simulink model "EDS"  (R2020a)
settings: Solver=VariableStepAuto  StartTime=0.0  StopTime=10.0  RelTol=1e-3
undefined symbols (not defined in the file): magnitude
libraries: simulink x2
settings Model: Creator=Administrator  LastModifiedBy=Administrator

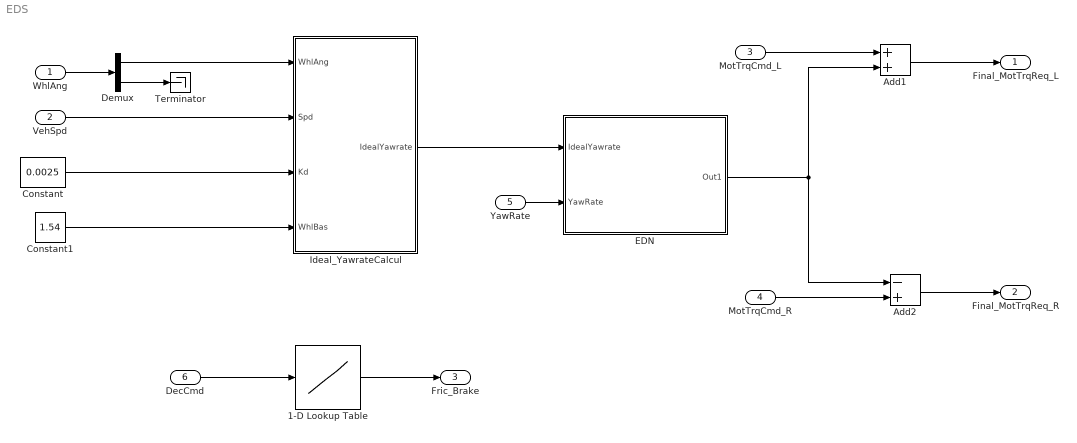
== system EDS ==
  WhlAng : Inport
  VehSpd : Inport  Port=2
  MotTrqCmd_L : Inport  Port=3
  MotTrqCmd_R : Inport  Port=4
  YawRate : Inport  Port=5
  DecCmd : Inport  Port=6
  1-D Lookup Table : Lookup_n-D  NumberOfTableDimensions=1  BreakpointsForDimension1=[0 , 0.2,0.4,0.6,0.8,1.0]  Table=[0 , 0.2,0.4,0.6,0.8,1.0]*60  InternalRulePriority=Speed  RndMeth=Simplest  InputSameDT=on
  Add1 : Sum
  Add2 : Sum  Inputs=-+
  Constant : Constant  Value=0.0025
  Constant1 : Constant  Value=1.54
  Demux : Demux  Outputs=2
  EDN : Subsystem
  Ideal_YawrateCalcul : Subsystem
  Terminator : Terminator
  Final_MotTrqReq_L : Outport
  Final_MotTrqReq_R : Outport  Port=2
  Fric_Brake : Outport  Port=3
  wires:
  WhlAng/1 -> Demux/1
  Demux/2 -> Terminator/1
  VehSpd/1 -> Ideal_YawrateCalcul/2(Spd)
  YawRate/1 -> EDN/2(YawRate)
  Add2/1 -> Final_MotTrqReq_R/1
  EDN/1(Out1) -> Add1/2, Add2/1
  MotTrqCmd_R/1 -> Add2/2
  Add1/1 -> Final_MotTrqReq_L/1
  MotTrqCmd_L/1 -> Add1/1
  Demux/1 -> Ideal_YawrateCalcul/1(WhlAng)
  Constant/1 -> Ideal_YawrateCalcul/3(Kd)
  Constant1/1 -> Ideal_YawrateCalcul/4(WhlBas)
  Ideal_YawrateCalcul/1(IdealYawrate) -> EDN/1(IdealYawrate)
  DecCmd/1 -> 1-D Lookup Table/1
  1-D Lookup Table/1 -> Fric_Brake/1

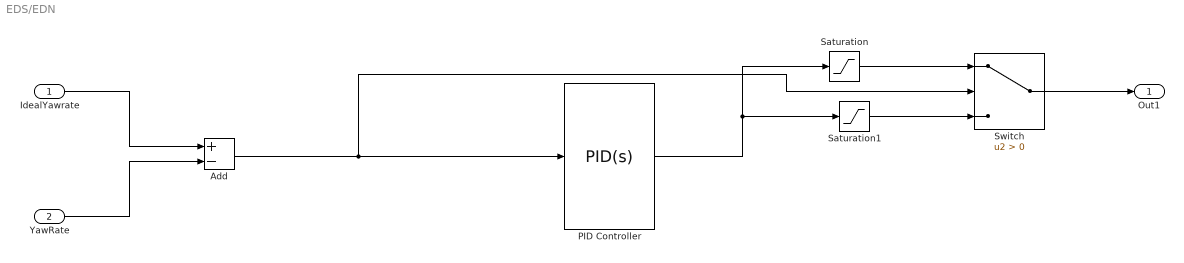
== system EDS/EDN ==
  IdealYawrate : Inport
  YawRate : Inport  Port=2
  Add : Sum  Inputs=+-
  PID Controller : simulink/Continuous/PID Controller  Controller=PID  Form=Parallel  TimeDomain=Continuous-time  UseExternalTs=off  SampleTime=-1  IntegratorMethod=Forward Euler  FilterMethod=Forward Euler  ControllerParametersSource=internal  P=2  I=1  D=0  UseFilter=on  N=100  TunerSelectOption=Transfer Function Based (PID Tuner App)  InitialConditionSource=internal  InitialConditionForIntegrator=0  InitialConditionForFilter=0  DifferentiatorICPrevScaledInput=0  ExternalReset=none  TrackingMode=off  Kt=1  LimitOutput=on  UpperSaturationLimit=30  LowerSaturationLimit=-30  LinearizeAsGain=on  AntiWindupMode=none  Kb=1  SaturateOnIntegerOverflow=on  POutMin=[]  POutMax=[]  IOutMin=[]  IOutMax=[]  DOutMin=[]  DOutMax=[]  NOutMin=[]  NOutMax=[]  SumOutMin=[]  SumOutMax=[]  SaturationOutMin=[]  SaturationOutMax=[]  PParamMin=[]  PParamMax=[]  IParamMin=[]  IParamMax=[]  DParamMin=[]  DParamMax=[]  NParamMin=[]  NParamMax=[]  KbParamMin=[]  KbParamMax=[]  KtParamMin=[]  KtParamMax=[]  KbOutMin=[]  KbOutMax=[]  KtOutMin=[]  KtOutMax=[]  IntegratorOutMin=[]  IntegratorOutMax=[]  FilterOutMin=[]  FilterOutMax=[]  SumI1OutMin=[]  SumI1OutMax=[]  SumI2OutMin=[]  SumI2OutMax=[]  SumI3OutMin=[]  SumI3OutMax=[]  SumI4OutMin=[]  SumI4OutMax=[]  SumDOutMin=[]  SumDOutMax=[]  DifferentiatorOutMin=[]  DifferentiatorOutMax=[]  FilterDiffOutCoefMin=[]  FilterDiffOutCoefMax=[]  ReciprocalOutMin=[]  ReciprocalOutMax=[]  SumDenOutMin=[]  SumDenOutMax=[]  SumNumOutMin=[]  SumNumOutMax=[]  DivideOutMin=[]  DivideOutMax=[]  UdiffTsProdOutMin=[]  UdiffTsProdOutMax=[]  NTsProdOutMin=[]  NTsProdOutMax=[]  UintegralTsProdOutMin=[]  UintegralTsProdOutMax=[]  UngainTsProdOutMin=[]  UngainTsProdOutMax=[]  IntegratorContinuousStateAttributes=''  IntegratorStateMustResolveToSignalObject=off  IntegratorRTWStateStorageClass=Auto  FilterContinuousStateAttributes=''  FilterStateMustResolveToSignalObject=off  FilterRTWStateStorageClass=Auto  ParallelPVariant=InternalParameters  IdealPVariant=Disabled  IVariant=InternalParameters  DVariant=InternalParameters  IntegratorVariant=Continuous  SatVariant=Enabled  AWVariant=Passthrough  PCopyVariant=Disabled  TRVariant=Disabled  FdbkBlocksVariant=Forward  IdealPFdbkVariant=Disabled  SatFdbkVariant=Disabled  DerivativeFilterVariant=ContFilter  NVariant=InternalParameters  NCopyVariant=Disabled  FilterICVariant=InternalICsFilter  IntegratorICVariant=InternalICs  ExternalResetVariant=Disabled  TRSumVariant=Passthrough  SumFdbkVariant=Disabled  SumVariant=Sum_PID  TsampFilterVariant=InternalTs  TsampNgainVariant=Passthrough  TsampIntegralVariant=Passthrough
  Saturation : Saturate  UpperLimit=inf  LowerLimit=0
  Saturation1 : Saturate  UpperLimit=0  LowerLimit=-inf
  Switch : Switch  Criteria=u2 > Threshold
  Out1 : Outport
  wires:
  Add/1 -> Switch/2, PID Controller/1
  Saturation/1 -> Switch/1
  Switch/1 -> Out1/1
  Saturation1/1 -> Switch/3
  YawRate/1 -> Add/2
  IdealYawrate/1 -> Add/1
  PID Controller/1 -> Saturation1/1, Saturation/1

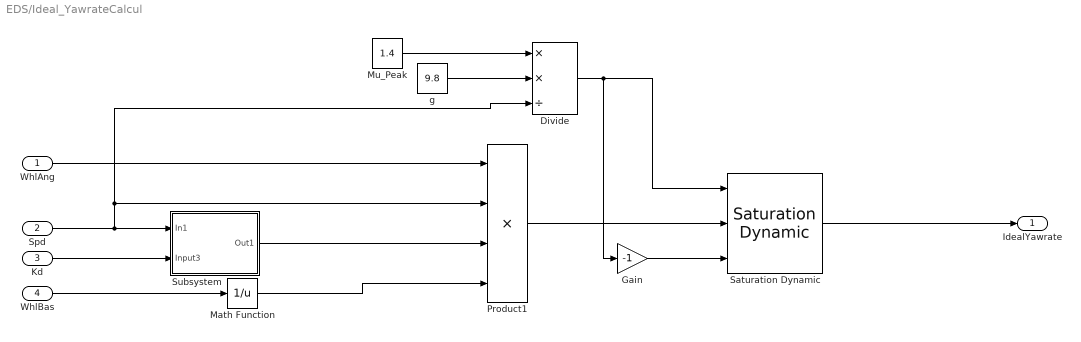
== system EDS/Ideal_YawrateCalcul ==
  WhlAng : Inport
  Spd : Inport  Port=2
  Kd : Inport  Port=3
  WhlBas : Inport  Port=4
  Divide : Product  Inputs=**/
  Gain : Gain  Gain=-1
  Math Function : Math  Operator=reciprocal  SaturateOnIntegerOverflow=on
  Mu_Peak : Constant  Value=1.4
  Product1 : Product  Inputs=4
  Saturation Dynamic : simulink/Discontinuities/Saturation Dynamic  OutMin=[]  OutMax=[]  OutDataTypeStr=Inherit: Same as second input  OutDataType=fixdt(1, 16)  OutScaling=2^-10  DoSatur=off
  Subsystem : Subsystem
  g : Constant  Value=9.8
  IdealYawrate : Outport
  wires:
  Spd/1 -> Divide/3, Product1/2, Subsystem/1(In1)
  Product1/1 -> Saturation Dynamic/2
  Divide/1 -> Gain/1, Saturation Dynamic/1
  g/1 -> Divide/2
  Mu_Peak/1 -> Divide/1
  Subsystem/1(Out1) -> Product1/3
  WhlAng/1 -> Product1/1
  Saturation Dynamic/1 -> IdealYawrate/1
  Gain/1 -> Saturation Dynamic/3
  WhlBas/1 -> Math Function/1
  Kd/1 -> Subsystem/2(Input3)
  Math Function/1 -> Product1/4

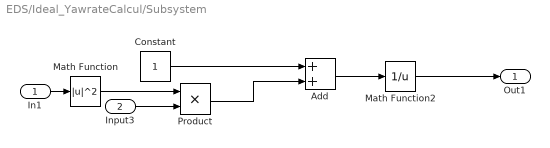
== system EDS/Ideal_YawrateCalcul/Subsystem ==
  In1 : Inport
  Input3 : Inport  Port=2
  Add : Sum
  Constant : Constant
  Math Function : Math  Operator=magnitude^2  SaturateOnIntegerOverflow=on
  Math Function2 : Math  Operator=reciprocal  SaturateOnIntegerOverflow=on
  Product : Product
  Out1 : Outport
  wires:
  Add/1 -> Math Function2/1
  Product/1 -> Add/2
  Input3/1 -> Product/2
  Math Function2/1 -> Out1/1
  Math Function/1 -> Product/1
  Constant/1 -> Add/1
  In1/1 -> Math Function/1
